simulink model "FOG_v8_1"  (R2023b)
settings: Solver=ode4  StartTime=0.0  StopTime=0.12  FixedStep=Ts_solver  RelTol=1e-3
undefined symbols (not defined in the file): a_aa, a_act, a_pi, actuator_cycles_before_reset, adc_sample_offset_s, b_aa, b_act, b_pi, depol_residual, eta_conn, eta_dep, eta_K1, eta_pol, f_mod, I_dark_A, K1_detector_ratio, K1_launch_ratio, K_norm_digital, K_phase_to_deg, K_ref, K_sag, K_sagnac_power, noise_enable, noise_sample_scale, Omega_feedback_limit_deg_s, Omega_step_final, Omega_step_time, P_source_W, phi0, pol_delta0_rad, pol_delta_amp_rad, pol_delta_freq_Hz, pol_delta_phase_rad, pol_enable, pol_nr_scale, pol_theta0_rad, pol_theta_amp_rad, pol_theta_freq_Hz, q_e, ref_delay_total_s, Rf, Rpd, seed_dark, seed_johnson, seed_opamp_en, seed_opamp_i, seed_photo, sigma_dark_sample_A, sigma_johnson_sample_A, sigma_opamp_current_sample_A, sigma_opamp_voltage_sample_A, slope_per_deg_s, sos_d, tau, Ts_adc, Ts_ctrl, Ts_noise, V_cal, Vadc_max, Vadc_min ... (+2)
settings Model: Creator=molik  LastModifiedBy=molik

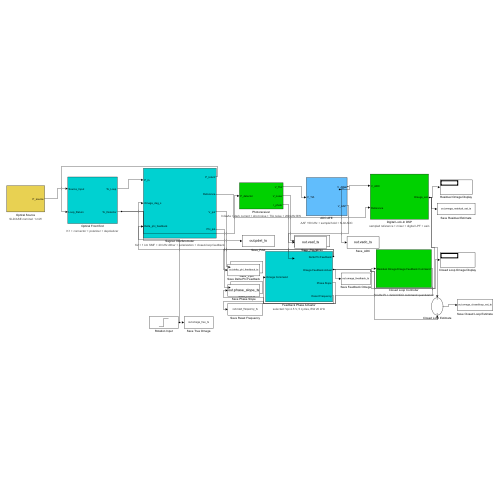
[thumbnail: Simulink's stored preview of the top-level diagram]
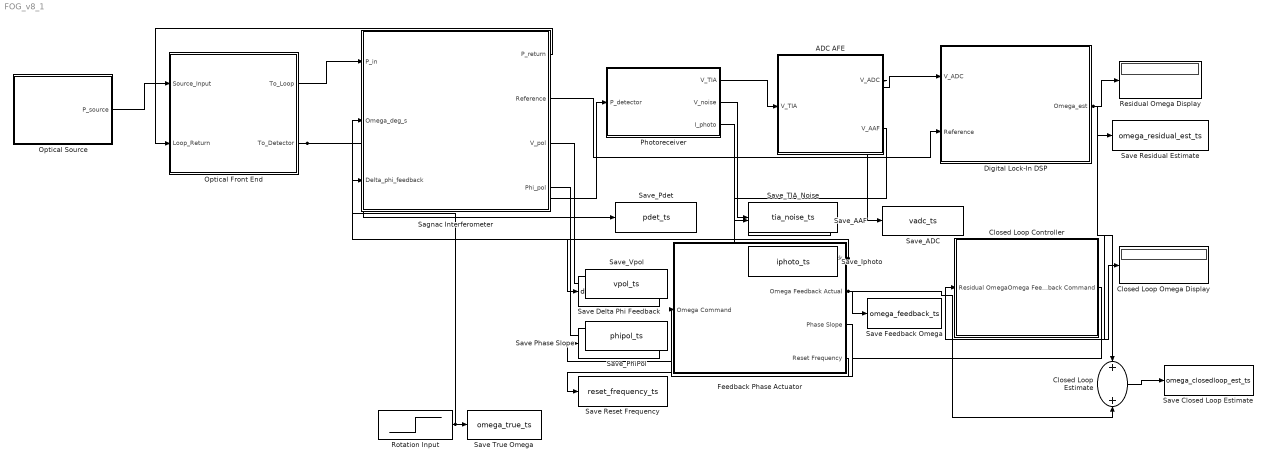
== system FOG_v8_1 ==
  ADC AFE : Subsystem
      settings: AttributesFormatString=AAF 150 kHz + sample/hold + N-bit ADC
  Closed Loop Controller : Subsystem
      settings: AttributesFormatString=10 kHz PI + 32-bit NCO command quantization
  Closed Loop Estimate : Sum
  Closed Loop Omega Display : Display
  Digital Lock-In DSP : Subsystem
      settings: AttributesFormatString=sampled reference + mixer + digital LPF + asin
  Feedback Phase Actuator : Subsystem
      settings: AttributesFormatString=selected: Vpi 4.5 V, 5 cycles, BW 20 kHz
  Optical Front End : Subsystem
      settings: AttributesFormatString=K1 + connector + polarizer + depolarizer
  Optical Source : Subsystem
      settings: AttributesFormatString=SLD/ASE nominal: 1 mW
  Photoreceiver : Subsystem
      settings: AttributesFormatString=InGaAs + dark current + shot noise + TIA noise + 200 kHz BW
  Residual Omega Display : Display
  Rotation Input : Step  Time=Omega_step_time  After=Omega_step_final  SampleTime=0
  Sagnac Interferometer : Subsystem
      settings: AttributesFormatString=K2 + 1 km SMF + 20 kHz dither + polarization + closed-loop feedback
  Save Closed Loop Estimate : ToWorkspace  VariableName=omega_closedloop_est_ts  SaveFormat=Timeseries  SampleTime=-1
  Save Delta Phi Feedback : ToWorkspace  VariableName=delta_phi_feedback_ts  SaveFormat=Timeseries  SampleTime=-1
  Save Feedback Omega : ToWorkspace  VariableName=omega_feedback_ts  SaveFormat=Timeseries  SampleTime=-1
  Save Phase Slope : ToWorkspace  VariableName=phase_slope_ts  SaveFormat=Timeseries  SampleTime=-1
  Save Reset Frequency : ToWorkspace  VariableName=reset_frequency_ts  SaveFormat=Timeseries  SampleTime=-1
  Save Residual Estimate : ToWorkspace  VariableName=omega_residual_est_ts  SaveFormat=Timeseries  SampleTime=-1
  Save True Omega : ToWorkspace  VariableName=omega_true_ts  SaveFormat=Timeseries  SampleTime=-1
  Save_AAF : ToWorkspace  VariableName=vaaf_ts  SaveFormat=Timeseries  SampleTime=-1
  Save_ADC : ToWorkspace  VariableName=vadc_ts  SaveFormat=Timeseries  SampleTime=-1
  Save_Iphoto : ToWorkspace  VariableName=iphoto_ts  SaveFormat=Timeseries  SampleTime=-1
  Save_Pdet : ToWorkspace  VariableName=pdet_ts  SaveFormat=Timeseries  SampleTime=-1
  Save_PhiPol : ToWorkspace  VariableName=phipol_ts  SaveFormat=Timeseries  SampleTime=-1
  Save_TIA_Noise : ToWorkspace  VariableName=tia_noise_ts  SaveFormat=Timeseries  SampleTime=-1
  Save_Vpol : ToWorkspace  VariableName=vpol_ts  SaveFormat=Timeseries  SampleTime=-1
  wires:
  Optical Source/1(P_source) -> Optical Front End/1(Source_Input)
  Optical Front End/2(To_Detector) -> Save_Pdet/1, Photoreceiver/1(P_detector)
  Photoreceiver/2(V_noise) -> Save_TIA_Noise/1
  Photoreceiver/3(I_photo) -> Save_Iphoto/1
  Photoreceiver/1(V_TIA) -> ADC AFE/1(V_TIA)
  ADC AFE/1(V_ADC) -> Digital Lock-In DSP/1(V_ADC), Save_ADC/1
  ADC AFE/2(V_AAF) -> Save_AAF/1
  Optical Front End/1(To_Loop) -> Sagnac Interferometer/1(P_in)
  Rotation Input/1 -> Sagnac Interferometer/2(Omega_deg_s), Save True Omega/1
  Sagnac Interferometer/1(P_return) -> Optical Front End/2(Loop_Return)
  Sagnac Interferometer/2(Reference) -> Digital Lock-In DSP/2(Reference)
  Sagnac Interferometer/3(V_pol) -> Save_Vpol/1
  Sagnac Interferometer/4(Phi_pol) -> Save_PhiPol/1
  Digital Lock-In DSP/1(Omega_est) -> Residual Omega Display/1, Save Residual Estimate/1, Closed Loop Controller/1(Residual Omega), Closed Loop Estimate/1
  Closed Loop Controller/1(Omega Feedback Command) -> Feedback Phase Actuator/1(Omega Command)
  Feedback Phase Actuator/2(Omega Feedback Actual) -> Closed Loop Omega Display/1, Save Feedback Omega/1, Closed Loop Estimate/2
  Feedback Phase Actuator/1(Delta Phi Feedback) -> Sagnac Interferometer/3(Delta_phi_feedback), Save Delta Phi Feedback/1
  Feedback Phase Actuator/3(Phase Slope) -> Save Phase Slope/1
  Feedback Phase Actuator/4(Reset Frequency) -> Save Reset Frequency/1
  Closed Loop Estimate/1 -> Save Closed Loop Estimate/1

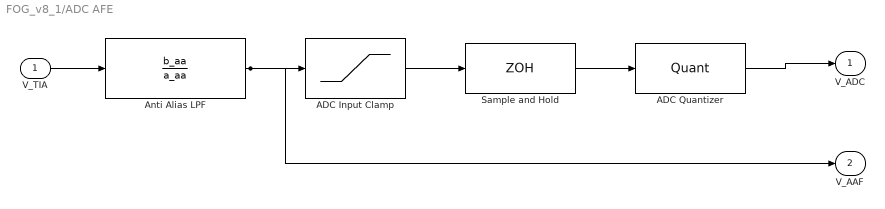
== system FOG_v8_1/ADC AFE ==
  V_TIA : Inport
  ADC Input Clamp : Saturate  UpperLimit=Vadc_max  LowerLimit=Vadc_min
  ADC Quantizer : Quantizer  QuantizationInterval=q_adc
  Anti Alias LPF : TransferFcn  Numerator=b_aa  Denominator=a_aa
  Sample and Hold : ZeroOrderHold  SampleTime=[Ts_adc adc_sample_offset_s]
  V_ADC : Outport
  V_AAF : Outport  Port=2
  wires:
  V_TIA/1 -> Anti Alias LPF/1
  Anti Alias LPF/1 -> ADC Input Clamp/1, V_AAF/1
  ADC Input Clamp/1 -> Sample and Hold/1
  Sample and Hold/1 -> ADC Quantizer/1
  ADC Quantizer/1 -> V_ADC/1

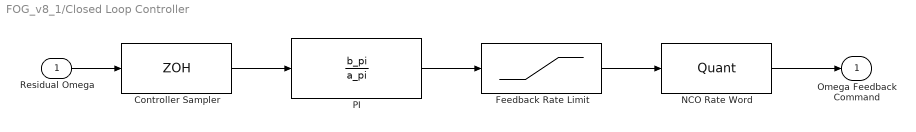
== system FOG_v8_1/Closed Loop Controller ==
  Residual Omega : Inport
  Controller Sampler : ZeroOrderHold  SampleTime=Ts_ctrl
  Feedback Rate Limit : Saturate  UpperLimit=Omega_feedback_limit_deg_s  LowerLimit=-Omega_feedback_limit_deg_s
  NCO Rate Word : Quantizer  QuantizationInterval=Omega_nco_LSB_deg_s
  PI : DiscreteTransferFcn  Numerator=b_pi  Denominator=a_pi  SampleTime=Ts_ctrl
  Omega Feedback Command : Outport
  wires:
  Residual Omega/1 -> Controller Sampler/1
  Controller Sampler/1 -> PI/1
  PI/1 -> Feedback Rate Limit/1
  Feedback Rate Limit/1 -> NCO Rate Word/1
  NCO Rate Word/1 -> Omega Feedback Command/1

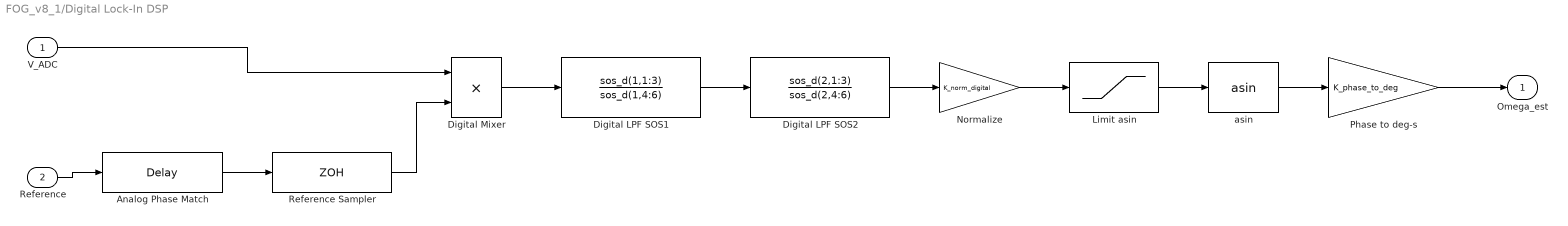
== system FOG_v8_1/Digital Lock-In DSP ==
  V_ADC : Inport
  Reference : Inport  Port=2
  Analog Phase Match : TransportDelay  DelayTime=ref_delay_total_s
  Digital LPF SOS1 : DiscreteTransferFcn  Numerator=sos_d(1,1:3)  Denominator=sos_d(1,4:6)  SampleTime=Ts_adc
  Digital LPF SOS2 : DiscreteTransferFcn  Numerator=sos_d(2,1:3)  Denominator=sos_d(2,4:6)  SampleTime=Ts_adc
  Digital Mixer : Product
  Limit asin : Saturate  UpperLimit=0.999999  LowerLimit=-0.999999
  Normalize : Gain  Gain=K_norm_digital
  Phase to deg-s : Gain  Gain=K_phase_to_deg
  Reference Sampler : ZeroOrderHold  SampleTime=[Ts_adc adc_sample_offset_s]
  asin : Trigonometry  Operator=asin
  Omega_est : Outport
  wires:
  V_ADC/1 -> Digital Mixer/1
  Reference/1 -> Analog Phase Match/1
  Analog Phase Match/1 -> Reference Sampler/1
  Reference Sampler/1 -> Digital Mixer/2
  Digital Mixer/1 -> Digital LPF SOS1/1
  Digital LPF SOS1/1 -> Digital LPF SOS2/1
  Digital LPF SOS2/1 -> Normalize/1
  Normalize/1 -> Limit asin/1
  Limit asin/1 -> asin/1
  asin/1 -> Phase to deg-s/1
  Phase to deg-s/1 -> Omega_est/1

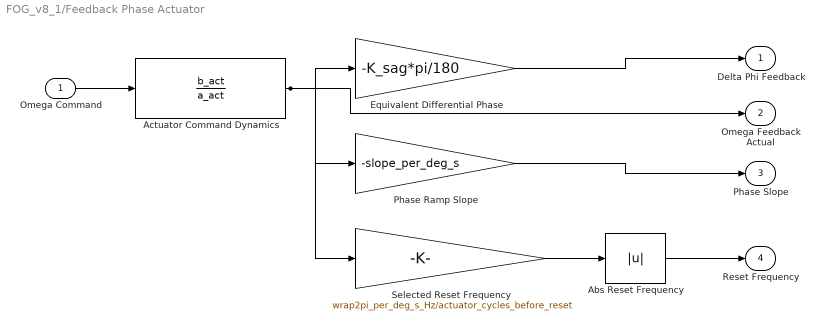
== system FOG_v8_1/Feedback Phase Actuator ==
  Omega Command : Inport
  Abs Reset Frequency : Abs  SaturateOnIntegerOverflow=off
  Actuator Command Dynamics : DiscreteTransferFcn  Numerator=b_act  Denominator=a_act  SampleTime=Ts_ctrl
  Equivalent Differential Phase : Gain  Gain=-K_sag*pi/180
  Phase Ramp Slope : Gain  Gain=-slope_per_deg_s
  Selected Reset Frequency : Gain  Gain=wrap2pi_per_deg_s_Hz/actuator_cycles_before_reset
  Delta Phi Feedback : Outport
  Omega Feedback Actual : Outport  Port=2
  Phase Slope : Outport  Port=3
  Reset Frequency : Outport  Port=4
  wires:
  Omega Command/1 -> Actuator Command Dynamics/1
  Actuator Command Dynamics/1 -> Equivalent Differential Phase/1, Omega Feedback Actual/1, Phase Ramp Slope/1, Selected Reset Frequency/1
  Equivalent Differential Phase/1 -> Delta Phi Feedback/1
  Phase Ramp Slope/1 -> Phase Slope/1
  Selected Reset Frequency/1 -> Abs Reset Frequency/1
  Abs Reset Frequency/1 -> Reset Frequency/1

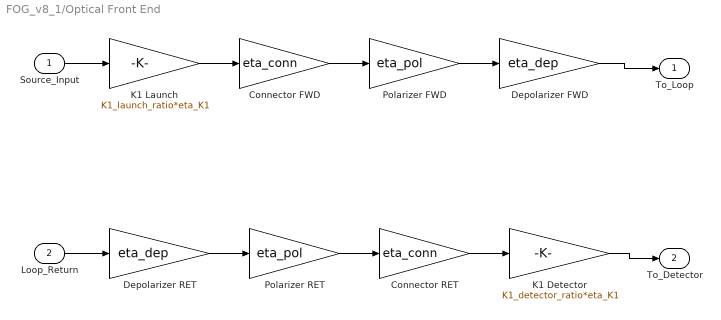
== system FOG_v8_1/Optical Front End ==
  Source_Input : Inport
  Loop_Return : Inport  Port=2
  Connector FWD : Gain  Gain=eta_conn
  Connector RET : Gain  Gain=eta_conn
  Depolarizer FWD : Gain  Gain=eta_dep
  Depolarizer RET : Gain  Gain=eta_dep
  K1 Detector : Gain  Gain=K1_detector_ratio*eta_K1
  K1 Launch : Gain  Gain=K1_launch_ratio*eta_K1
  Polarizer FWD : Gain  Gain=eta_pol
  Polarizer RET : Gain  Gain=eta_pol
  To_Loop : Outport
  To_Detector : Outport  Port=2
  wires:
  Source_Input/1 -> K1 Launch/1
  K1 Launch/1 -> Connector FWD/1
  Connector FWD/1 -> Polarizer FWD/1
  Polarizer FWD/1 -> Depolarizer FWD/1
  Depolarizer FWD/1 -> To_Loop/1
  Loop_Return/1 -> Depolarizer RET/1
  Depolarizer RET/1 -> Polarizer RET/1
  Polarizer RET/1 -> Connector RET/1
  Connector RET/1 -> K1 Detector/1
  K1 Detector/1 -> To_Detector/1

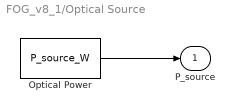
== system FOG_v8_1/Optical Source ==
  Optical Power : Constant  Value=P_source_W
  P_source : Outport
  wires:
  Optical Power/1 -> P_source/1

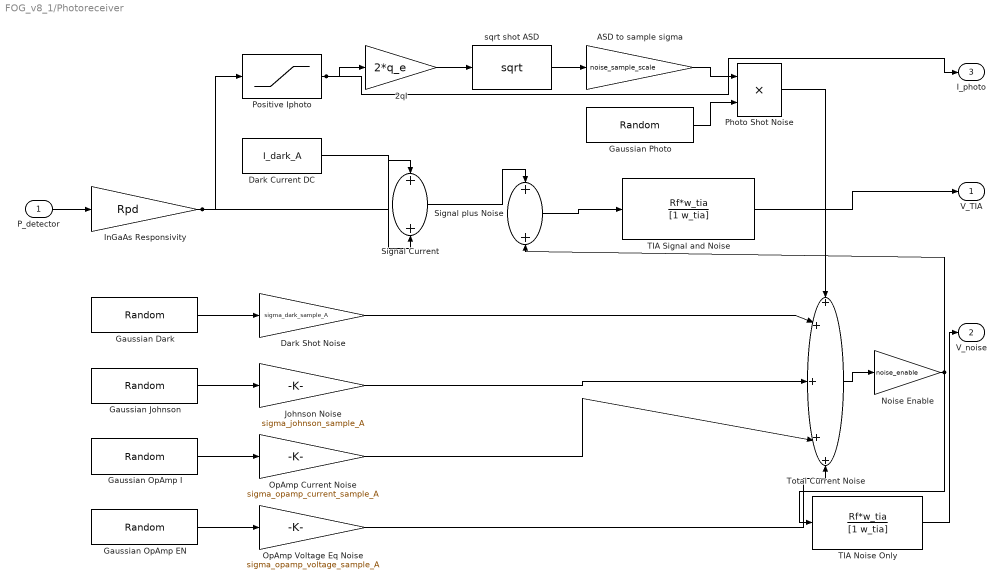
== system FOG_v8_1/Photoreceiver ==
  P_detector : Inport
  2qI : Gain  Gain=2*q_e
  ASD to sample sigma : Gain  Gain=noise_sample_scale
  Dark Current DC : Constant  Value=I_dark_A
  Dark Shot Noise : Gain  Gain=sigma_dark_sample_A
  Gaussian Dark : RandomNumber  Seed=seed_dark  SampleTime=Ts_noise
  Gaussian Johnson : RandomNumber  Seed=seed_johnson  SampleTime=Ts_noise
  Gaussian OpAmp EN : RandomNumber  Seed=seed_opamp_en  SampleTime=Ts_noise
  Gaussian OpAmp I : RandomNumber  Seed=seed_opamp_i  SampleTime=Ts_noise
  Gaussian Photo : RandomNumber  Seed=seed_photo  SampleTime=Ts_noise
  InGaAs Responsivity : Gain  Gain=Rpd
  Johnson Noise : Gain  Gain=sigma_johnson_sample_A
  Noise Enable : Gain  Gain=noise_enable
  OpAmp Current Noise : Gain  Gain=sigma_opamp_current_sample_A
  OpAmp Voltage Eq Noise : Gain  Gain=sigma_opamp_voltage_sample_A
  Photo Shot Noise : Product
  Positive Iphoto : Saturate  UpperLimit=inf  LowerLimit=0
  Signal Current : Sum
  Signal plus Noise : Sum
  TIA Noise Only : TransferFcn  Numerator=Rf*w_tia  Denominator=[1 w_tia]
  TIA Signal and Noise : TransferFcn  Numerator=Rf*w_tia  Denominator=[1 w_tia]
  Total Current Noise : Sum  Inputs=+++++
  sqrt shot ASD : Math  Operator=sqrt
  V_TIA : Outport
  V_noise : Outport  Port=2
  I_photo : Outport  Port=3
  wires:
  Gaussian Dark/1 -> Dark Shot Noise/1
  Gaussian Johnson/1 -> Johnson Noise/1
  Gaussian OpAmp I/1 -> OpAmp Current Noise/1
  Gaussian OpAmp EN/1 -> OpAmp Voltage Eq Noise/1
  P_detector/1 -> InGaAs Responsivity/1
  InGaAs Responsivity/1 -> Signal Current/1, Positive Iphoto/1
  Dark Current DC/1 -> Signal Current/2
  Signal Current/1 -> Signal plus Noise/1
  Noise Enable/1 -> Signal plus Noise/2, TIA Noise Only/1
  Signal plus Noise/1 -> TIA Signal and Noise/1
  TIA Signal and Noise/1 -> V_TIA/1
  Positive Iphoto/1 -> 2qI/1, I_photo/1
  2qI/1 -> sqrt shot ASD/1
  sqrt shot ASD/1 -> ASD to sample sigma/1
  ASD to sample sigma/1 -> Photo Shot Noise/1
  Gaussian Photo/1 -> Photo Shot Noise/2
  Photo Shot Noise/1 -> Total Current Noise/1
  Dark Shot Noise/1 -> Total Current Noise/2
  Johnson Noise/1 -> Total Current Noise/3
  OpAmp Current Noise/1 -> Total Current Noise/4
  OpAmp Voltage Eq Noise/1 -> Total Current Noise/5
  Total Current Noise/1 -> Noise Enable/1
  TIA Noise Only/1 -> V_noise/1

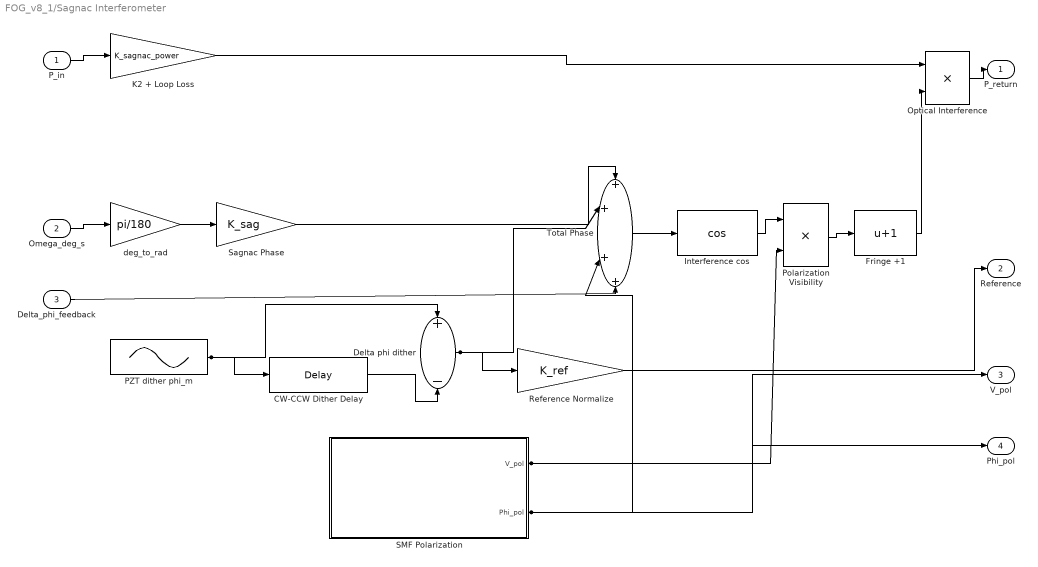
== system FOG_v8_1/Sagnac Interferometer ==
  P_in : Inport
  Omega_deg_s : Inport  Port=2
  Delta_phi_feedback : Inport  Port=3
  CW-CCW Dither Delay : TransportDelay  DelayTime=tau
  Delta phi dither : Sum  Inputs=+-
  Fringe +1 : Bias  Bias=1  SaturateOnIntegerOverflow=off
  Interference cos : Trigonometry  Operator=cos
  K2 + Loop Loss : Gain  Gain=K_sagnac_power
  Optical Interference : Product
  PZT dither phi_m : Sin  Amplitude=phi0  Frequency=2*pi*f_mod  SampleTime=0
  Polarization Visibility : Product
  Reference Normalize : Gain  Gain=K_ref
  SMF Polarization : Subsystem
  Sagnac Phase : Gain  Gain=K_sag
  Total Phase : Sum  Inputs=++++
  deg_to_rad : Gain  Gain=pi/180
  P_return : Outport
  Reference : Outport  Port=2
  V_pol : Outport  Port=3
  Phi_pol : Outport  Port=4
  wires:
  P_in/1 -> K2 + Loop Loss/1
  K2 + Loop Loss/1 -> Optical Interference/1
  Omega_deg_s/1 -> deg_to_rad/1
  deg_to_rad/1 -> Sagnac Phase/1
  Sagnac Phase/1 -> Total Phase/1
  PZT dither phi_m/1 -> Delta phi dither/1, CW-CCW Dither Delay/1
  CW-CCW Dither Delay/1 -> Delta phi dither/2
  Delta phi dither/1 -> Total Phase/2, Reference Normalize/1
  SMF Polarization/2(Phi_pol) -> Total Phase/3, Phi_pol/1
  Delta_phi_feedback/1 -> Total Phase/4
  Total Phase/1 -> Interference cos/1
  Interference cos/1 -> Polarization Visibility/1
  SMF Polarization/1(V_pol) -> Polarization Visibility/2, V_pol/1
  Polarization Visibility/1 -> Fringe +1/1
  Fringe +1/1 -> Optical Interference/2
  Optical Interference/1 -> P_return/1
  Reference Normalize/1 -> Reference/1

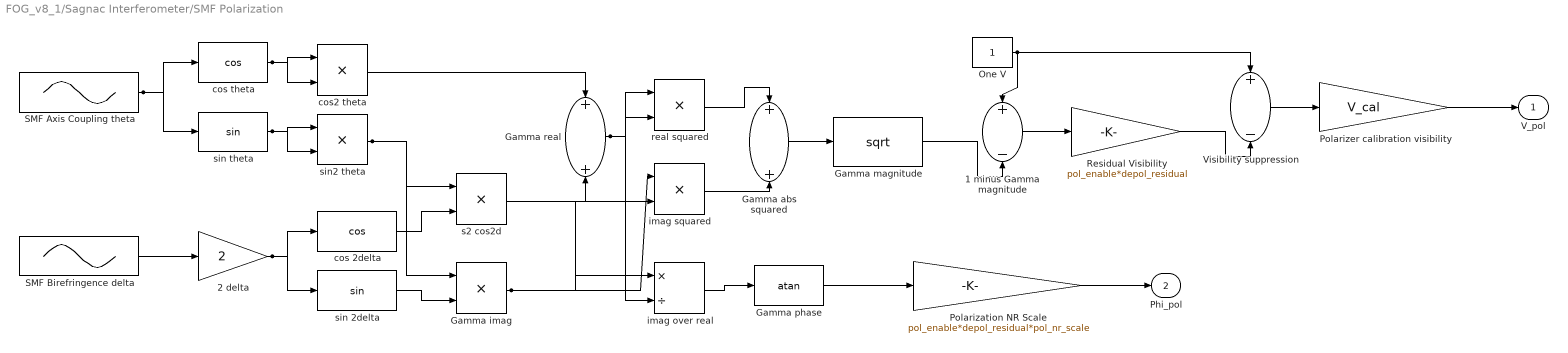
== system FOG_v8_1/Sagnac Interferometer/SMF Polarization ==
  1 minus Gamma magnitude : Sum  Inputs=+-
  2 delta : Gain  Gain=2
  Gamma abs squared : Sum
  Gamma imag : Product
  Gamma magnitude : Math  Operator=sqrt
  Gamma phase : Trigonometry  Operator=atan
  Gamma real : Sum
  One V : Constant
  Polarization NR Scale : Gain  Gain=pol_enable*depol_residual*pol_nr_scale
  Polarizer calibration visibility : Gain  Gain=V_cal
  Residual Visibility : Gain  Gain=pol_enable*depol_residual
  SMF Axis Coupling theta : Sin  Amplitude=pol_theta_amp_rad  Bias=pol_theta0_rad  Frequency=2*pi*pol_theta_freq_Hz  SampleTime=0
  SMF Birefringence delta : Sin  Amplitude=pol_delta_amp_rad  Bias=pol_delta0_rad  Frequency=2*pi*pol_delta_freq_Hz  Phase=pol_delta_phase_rad  SampleTime=0
  Visibility suppression : Sum  Inputs=+-
  cos 2delta : Trigonometry  Operator=cos
  cos theta : Trigonometry  Operator=cos
  cos2 theta : Product
  imag over real : Product  Inputs=*/
  imag squared : Product
  real squared : Product
  s2 cos2d : Product
  sin 2delta : Trigonometry
  sin theta : Trigonometry
  sin2 theta : Product
  V_pol : Outport
  Phi_pol : Outport  Port=2
  wires:
  SMF Axis Coupling theta/1 -> cos theta/1, sin theta/1
  cos theta/1 -> cos2 theta/1, cos2 theta/2
  sin theta/1 -> sin2 theta/1, sin2 theta/2
  SMF Birefringence delta/1 -> 2 delta/1
  2 delta/1 -> cos 2delta/1, sin 2delta/1
  sin2 theta/1 -> s2 cos2d/1, Gamma imag/1
  cos 2delta/1 -> s2 cos2d/2
  cos2 theta/1 -> Gamma real/1
  s2 cos2d/1 -> Gamma real/2
  sin 2delta/1 -> Gamma imag/2
  Gamma real/1 -> real squared/1, real squared/2, imag over real/2
  Gamma imag/1 -> imag squared/1, imag squared/2, imag over real/1
  real squared/1 -> Gamma abs squared/1
  imag squared/1 -> Gamma abs squared/2
  Gamma abs squared/1 -> Gamma magnitude/1
  imag over real/1 -> Gamma phase/1
  Gamma phase/1 -> Polarization NR Scale/1
  One V/1 -> 1 minus Gamma magnitude/1, Visibility suppression/1
  Gamma magnitude/1 -> 1 minus Gamma magnitude/2
  1 minus Gamma magnitude/1 -> Residual Visibility/1
  Residual Visibility/1 -> Visibility suppression/2
  Visibility suppression/1 -> Polarizer calibration visibility/1
  Polarizer calibration visibility/1 -> V_pol/1
  Polarization NR Scale/1 -> Phi_pol/1
